simulink model "Model_1_4_zawieszenia"  (R2024b)
settings: Solver=ode4  StartTime=0.0  StopTime=20  FixedStep=0.001  RelTol=1e-3
undefined symbols (not defined in the file): b1, b2, k1, k2, m1, m2
settings Model: Creator=mati  LastModifiedBy=mati

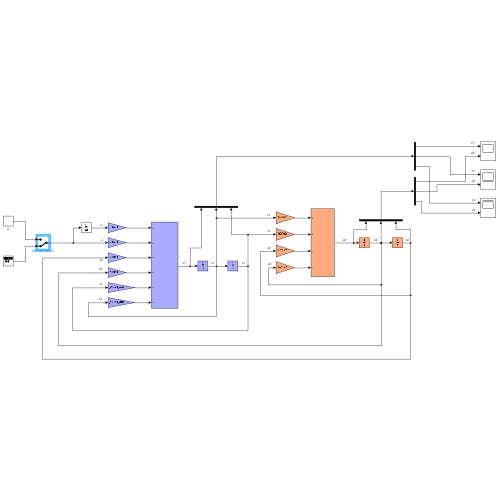
[thumbnail: Simulink's stored preview of the top-level diagram]
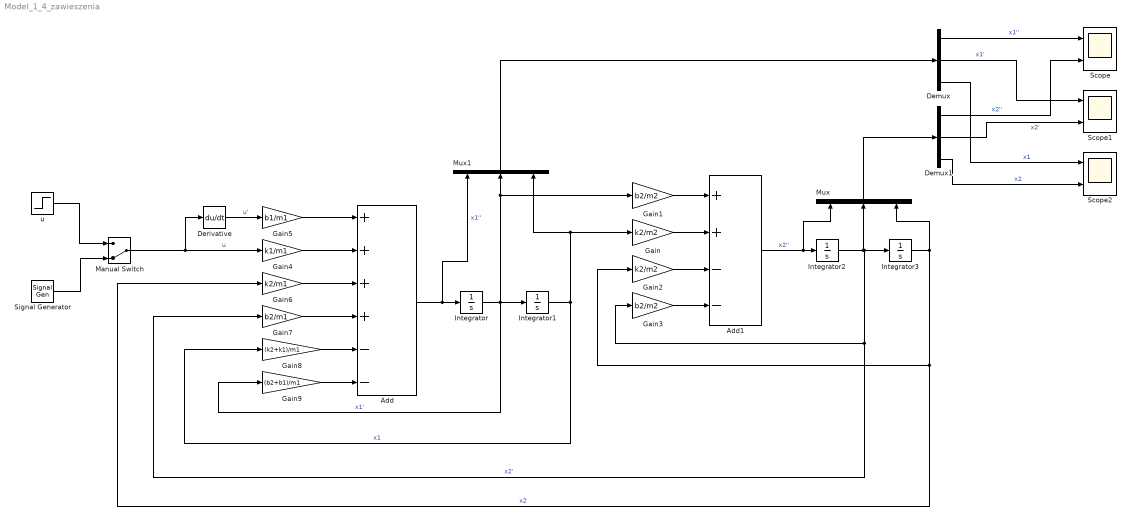
== system Model_1_4_zawieszenia ==
  Add : Sum  Inputs=++++--
  Add1 : Sum  Inputs=++--
  Demux : Demux  Outputs=3
  Demux1 : Demux  Outputs=3
  Derivative : Derivative
  Gain : Gain  Gain=k2/m2
  Gain1 : Gain  Gain=b2/m2
  Gain2 : Gain  Gain=k2/m2
  Gain3 : Gain  Gain=b2/m2
  Gain4 : Gain  Gain=k1/m1
  Gain5 : Gain  Gain=b1/m1
  Gain6 : Gain  Gain=k2/m1
  Gain7 : Gain  Gain=b2/m1
  Gain8 : Gain  Gain=(k2+k1)/m1
  Gain9 : Gain  Gain=(b2+b1)/m1
  Integrator{,1..3} (4 alike) : Integrator
  Manual Switch : ManualSwitch  CurrentSetting=0
  Mux : Mux  Inputs=3
  Mux1 : Mux  Inputs=3
  Scope : Scope  NumInputPorts=2
  Scope1 : Scope  NumInputPorts=2
  Scope2 : Scope  NumInputPorts=2
  Signal Generator : SignalGenerator  WaveForm=square  Amplitude=0.1  Frequency=0.5  Units=rad/sec
  u : Step  SampleTime=0
  wires:
  Add/1 -> Mux1/1, Integrator/1  "x1''"
  Integrator/1 -> Gain9/1, Integrator1/1, Gain1/1, Mux1/2  "x1'"
  Integrator1/1 -> Gain8/1, Gain/1, Mux1/3  "x1"
  Add1/1 -> Mux/1, Integrator2/1  "x2''"
  Integrator2/1 -> Integrator3/1, Gain7/1, Gain3/1, Mux/2  "x2'"
  Gain/1 -> Add1/2
  Integrator3/1 -> Gain6/1, Gain2/1, Mux/3  "x2"
  Signal Generator/1 -> Manual Switch/2
  u/1 -> Manual Switch/1
  Manual Switch/1 -> Derivative/1, Gain4/1  "u"
  Gain1/1 -> Add1/1
  Gain2/1 -> Add1/3
  Gain3/1 -> Add1/4
  Gain4/1 -> Add/2
  Gain9/1 -> Add/6
  Gain8/1 -> Add/5
  Gain7/1 -> Add/4
  Gain6/1 -> Add/3
  Gain5/1 -> Add/1
  Mux/1 -> Demux1/1
  Derivative/1 -> Gain5/1  "u'"
  Mux1/1 -> Demux/1
  Demux/2 -> Scope1/1  "x1'"
  Demux/1 -> Scope/1  "x1''"
  Demux1/1 -> Scope/2  "x2''"
  Demux1/2 -> Scope1/2  "x2'"
  Demux/3 -> Scope2/1  "x1"
  Demux1/3 -> Scope2/2  "x2"
